simulink model "Simulation"  (R2020b)
settings: Solver=VariableStepAuto  StartTime=0.0  StopTime=10  RelTol=1e-3
undefined symbols (not defined in the file): Controller_Mode, DiscIntNeverNeededParam, InitalDroneXYZ, maxOmega, plant_N, ts_camera, ts_control
libraries: simulink x4, sim3dcameralib x3, uavsim3dlib x2, dspfdesign x1, rllib x1, deeplib x1, visiongeotforms x1, sim3dlib x1
settings Model: DataDictionary=Dictionary.sldd  EnableAccessToBaseWorkspace=off  VariantFading=off  OrderedModelArguments=off  Creator=elbit  LastModifiedBy=elbit
settings DebuggingCC: BusObjectLabelMismatch=error

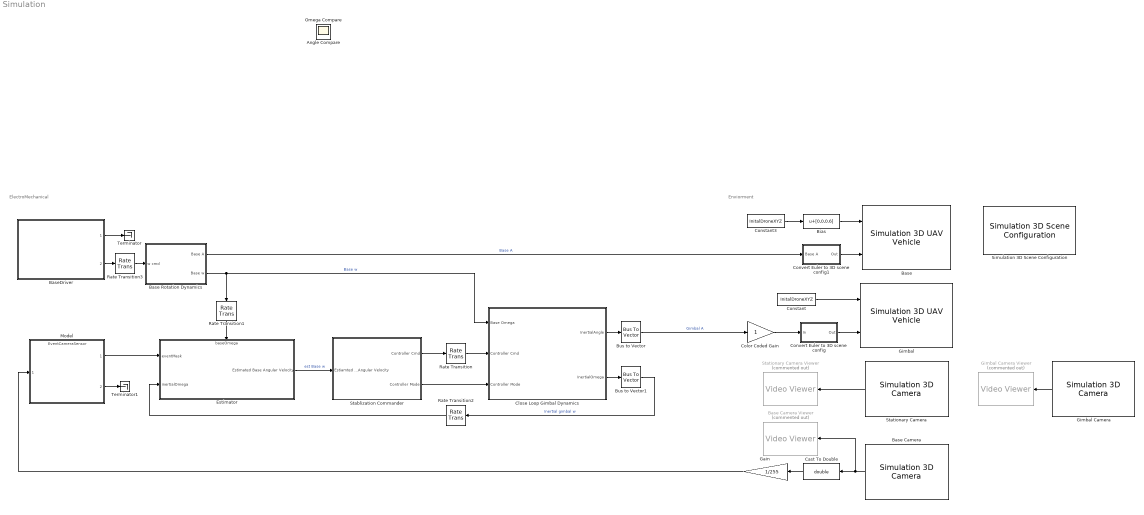
== system Simulation ==
  note: ElectroMechanical
  note: Enviorment
  Base : uavsim3dlib/Simulation 3D UAV Vehicle  Mesh=Quadrotor  Color=Black  ActorName=Base  InitialTranslation=InitalDroneXYZ  InitialRotation=[0 0 0]  SampleTime=-1  ActorType=SimulinkVehicle  ID=C  aMode=4  ActorTag=Base
      settings: SourceProductName=UAV Toolbox
  Base Camera : sim3dcameralib/Simulation 3D Camera  Priority=1  sensorTag=Sim3dSensor1  sensorId=1  sensorName=Sim3dSensor1  vehTagList={'Base';'Gimbal';'Scene Origin'}  vehTag=Base  mountLoc=Origin  offsetFlag=on  tmountOffset=[0.1, 0, 0]  rmountOffset=[0, 0, 0]  FocalLength=[1109, 1109]  OpticalCenter=[640, 360]  ImageSize=[720, 1280]  RadialDistortion=[0, 0]  TangentialDistortion=[0, 0]  SensorSkew=0  DepthOutportEnabled=off  SemanticOutportEnabled=off  TransformOutportEnabled=off  SampleTime=-1  mountPoint=[0.1 0 0]  mountOrientation=[0 0 0]  aMode=4  ID=1
      settings: SourceProductBaseCode=DR,UV,VE
  Base Camera Viewer : VideoViewer  Commented=on  FigPos=[2450.6 616.4 417.6 316]
  Base Rotation Dynamics : Subsystem  TreatAsAtomicUnit=on
  BaseDriver : Subsystem  TreatAsAtomicUnit=on  ReferencedSubsystem=BaseDriver
  Bias : Bias  Bias=[0,0,0.6]
  Bus to Vector : BusToVector
  Bus to Vector1 : BusToVector
  Cast To Double : DataTypeConversion  OutDataTypeStr=double
  Close Loop Gimbal Dynamics : Subsystem
  Color Coded Gain : Gain  OutDataTypeStr=Inherit: Same as input
      settings: OpenFcn=|
      | if get_param(gcbh,'gain')-48 set_param(gcbh,'gain','0','backgroundcolor','red');
      | else set_param(gcbh,'gain','1','backgroundcolor','green');
      | end
  Constant : Constant  Value=InitalDroneXYZ
  Constant3 : Constant  Value=InitalDroneXYZ
  Convert Euler to 3D scene config : Subsystem
  Convert Euler to 3D scene config1 : Subsystem
  Estimator : Subsystem  Variant=on  VariantControlMode=label  VariantControl=Choice  LabelModeActiveChoice=RNN
      settings: PortSchema="{\"entries\":[{\"content\":{\"sides\":[{\"content\":{\"connectorIds\":[\"In1\",\"In2\"]},\"type\":\"ConnectorPlacement.EquallySpacedRectSide\",\"uuid\":\"14ed0ca0-4e82-4a39-abac-b2cc8c23d388\"},{\"content\":{\"connectorIds\":[\"Out1\"],\"side\":\"RIGHT\"},\"type\":\"ConnectorPlacement.EquallySpacedRectSide\",\"uuid\":\"e489f507-16a0-46e9-ac1f-44f6d2c4c602\"},{\"content\":{\"connectorIds\":[\"In3\"],\"side\":\"TOP\"},\"type\":\"ConnectorPlacement.EquallySpacedRectSide\",\"uuid\":\"bc2047a9-ba61-4167-bd93-99be29e3b1d9\"},{\"content\":{\"connectorIds\":[],\"side\":\"HIDDEN\"},\"type\":\"ConnectorPlacement.EquallySpacedRectSide\",\"uuid\":\"51c71e1a-03eb-448f-a426-a7c596e1bf88\"}]},\"type\":\"ConnectorPlacement.EquallySpacedConnector\",\"uuid\":\"2c590113-b0cf-4c4b-9d58-bf60918ff368\"}],\"packageUris\":[\"http://schema.mathworks.com/mf0/Connector/R2020b\"],\"version\":\"1.0\"}"
  Gain : Gain  Gain=1/255
  Gimbal : uavsim3dlib/Simulation 3D UAV Vehicle  Mesh=Quadrotor  Color=Black  ActorName=Gimbal  InitialTranslation=InitalDroneXYZ  InitialRotation=[0 0 0]  SampleTime=-1  ActorType=SimulinkVehicle  ID=C  aMode=4  ActorTag=Gimbal
      settings: SourceProductName=UAV Toolbox
  Gimbal Camera : sim3dcameralib/Simulation 3D Camera  Priority=1  sensorTag=Sim3dSensor3  sensorId=3  sensorName=Sim3dSensor3  vehTagList={'Base';'Gimbal';'Scene Origin'}  vehTag=Gimbal  mountLoc=Origin  offsetFlag=on  tmountOffset=[0.1, 0, 0]  rmountOffset=[0, 0, 0]  FocalLength=[1109, 1109]  OpticalCenter=[640, 360]  ImageSize=[720, 1280]  RadialDistortion=[0, 0]  TangentialDistortion=[0, 0]  SensorSkew=0  DepthOutportEnabled=off  SemanticOutportEnabled=off  TransformOutportEnabled=off  SampleTime=-1  mountPoint=[0.1 0 0]  mountOrientation=[0 0 0]  aMode=4  ID=3
      settings: SourceProductBaseCode=DR,UV,VE
  Gimbal Camera Viewer : VideoViewer  Commented=on  FigPos=[125.8 875.6 524.8 320.8]
  Model : ModelReference  ModelNameDialog=EventCameraSensor.slx  ModelReferenceVersion=1.37
  Rate Transition : RateTransition  OutPortSampleTime=ts_control
  Rate Transition1 : RateTransition  OutPortSampleTime=ts_camera
  Rate Transition2 : RateTransition
  Rate Transition3 : RateTransition
  Simulation 3D Scene Configuration : sim3dlib/Simulation 3D Scene Configuration  Priority=0  ProjectFormat=Default Scenes  SceneDesc=US city block  ProjectName=MathWorks_Aerospace.exe  ScenePath=/Game/Maps/USCityBlock  vehTagList={'Base';'Gimbal';'Scene Origin'}  vehTag=Scene Origin  OpVisEn=off  Ts=ts_camera  EnableWindow=off  sensorTag=MainCamera1  sensorId=1  sensorName=MainCamera1  mountLoc=Origin  offsetFlag=off  tmountOffset=[0, 0, 0]  rmountOffset=[0, 0, 0]  HorizontalResolution=1280  VerticalResolution=720  HorizontalFOV=60  mountPoint=[0 0 0]  mountOrientation=[0 0 0]  aMode=4  ID=1
      settings: SourceProductBaseCode=DR,UV,VE
  Stablization Commander : Subsystem  TreatAsAtomicUnit=on
  Stationary Camera : sim3dcameralib/Simulation 3D Camera  Priority=1  sensorTag=Sim3dSensor2  sensorId=2  sensorName=Sim3dSensor2  vehTagList={'Base';'Gimbal';'Scene Origin'}  vehTag=Scene Origin  mountLoc=Origin  offsetFlag=on  tmountOffset=[10.88,83.6,8.181]  rmountOffset=[0,0.1047,-2.34]*180/pi  FocalLength=[1109, 1109]  OpticalCenter=[640, 360]  ImageSize=[720, 1280]  RadialDistortion=[0, 0]  TangentialDistortion=[0, 0]  SensorSkew=0  DepthOutportEnabled=off  SemanticOutportEnabled=off  TransformOutportEnabled=off  SampleTime=-1  mountPoint=[10.88 -83.6 8.181]  mountOrientation=[0 -5.99886811501972 134.072124060613]  aMode=4  ID=2
      settings: SourceProductBaseCode=DR,UV,VE
  Stationary Camera Viewer : VideoViewer  Commented=on  FigPos=[1048.2 851.6 517.6 520]
  Terminator : Terminator
  Terminator1 : Terminator
  Angle Compare : Scope
  Omega Compare : Scope
  wires:
  Constant/1 -> Gimbal/1
  Base Camera/1 -> Base Camera Viewer/1, Cast To Double/1
  Model/2 -> Terminator1/1
  Close Loop Gimbal Dynamics/1(InertialAngle) -> Bus to Vector/1
  Close Loop Gimbal Dynamics/2(InertialOmega) -> Bus to Vector1/1
  Cast To Double/1 -> Gain/1
  Gain/1 -> Model/1
  Bus to Vector/1 -> Color Coded Gain/1  "Gimbal A"
  Color Coded Gain/1 -> Convert Euler to 3D scene config/1(In)
  Stablization Commander/2(Controller Mode) -> Close Loop Gimbal Dynamics/3(Controller Mode)
  Stationary Camera/1 -> Stationary Camera Viewer/1
  Convert Euler to 3D scene config/1(Out) -> Gimbal/2
  Rate Transition1/1 -> Estimator/3(baseOmega)
  Rate Transition/1 -> Close Loop Gimbal Dynamics/2(Controller Cmd)
  Stablization Commander/1(Controller Cmd) -> Rate Transition/1
  Convert Euler to 3D scene config1/1(Out) -> Base/2
  Constant3/1 -> Bias/1
  Base Rotation Dynamics/1(Base A) -> Convert Euler to 3D scene config1/1(Base A)  "Base A"
  Bus to Vector1/1 -> Rate Transition2/1  "Inertial gimbal w"
  Bias/1 -> Base/1
  BaseDriver/2 -> Rate Transition3/1
  BaseDriver/1 -> Terminator/1
  Model/1 -> Estimator/1(eventMask)
  Base Rotation Dynamics/2(Base w) -> Close Loop Gimbal Dynamics/1(Base Omega), Rate Transition1/1  "Base w"
  Gimbal Camera/1 -> Gimbal Camera Viewer/1
  Rate Transition2/1 -> Estimator/2(inertialOmega)
  Rate Transition3/1 -> Base Rotation Dynamics/1(w cmd)
  Estimator/1(Estimated Base Angular Velocity) -> Stablization Commander/1(Estiamted Base Angular Velocity)  "est Base w"

== system Simulation/Base Rotation Dynamics ==
  w cmd : Inport
  Demux : Demux  Outputs=3
  Mux : Mux  Inputs=3
  RotationIntegrator : Integrator  InitialCondition=[0 0 0]
  Transfer Fcn : TransferFcn  Numerator=(2*pi*7)^2  Denominator=[1,2*1*(2*pi*7),(2*pi*7)^2]
  Transfer Fcn1 : TransferFcn  Numerator=(2*pi*7)^2  Denominator=[1,2*1*(2*pi*7),(2*pi*7)^2]
  Transfer Fcn2 : TransferFcn  Numerator=(2*pi*7)^2  Denominator=[1,2*1*(2*pi*7),(2*pi*7)^2]
  Base A : Outport
  Base w : Outport  Port=2
  wires:
  Demux/3 -> Transfer Fcn2/1
  Demux/2 -> Transfer Fcn1/1
  RotationIntegrator/1 -> Base A/1
  w cmd/1 -> Demux/1
  Mux/1 -> Base w/1, RotationIntegrator/1
  Transfer Fcn2/1 -> Mux/3
  Transfer Fcn1/1 -> Mux/2
  Transfer Fcn/1 -> Mux/1
  Demux/1 -> Transfer Fcn/1

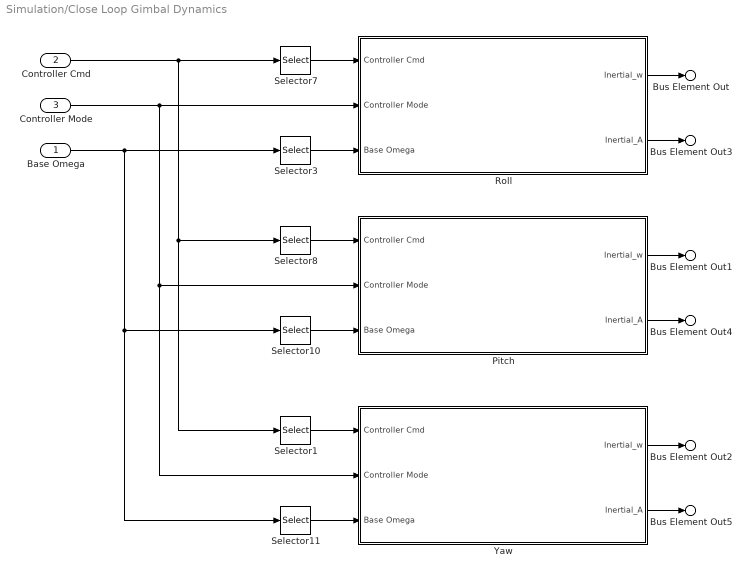
== system Simulation/Close Loop Gimbal Dynamics ==
  Base Omega : Inport
  Controller Cmd : Inport  Port=2
  Controller Mode : Inport  Port=3
  Pitch : Subsystem  Variant=on  VariantControlMode=label  VariantControl=Choice  LabelModeActiveChoice=Simple
  Roll : Subsystem  Variant=on  VariantControlMode=label  VariantControl=Choice  LabelModeActiveChoice=Simple
  Selector1 : Selector  InputPortWidth=3  IndexOptions=Index vector (dialog)  Indices=3  OutputSizes=1
  Selector10 : Selector  InputPortWidth=3  IndexOptions=Index vector (dialog)  Indices=2  OutputSizes=1
  Selector11 : Selector  InputPortWidth=3  IndexOptions=Index vector (dialog)  Indices=3  OutputSizes=1
  Selector3 : Selector  InputPortWidth=3  IndexOptions=Index vector (dialog)  Indices=1  OutputSizes=1
  Selector7 : Selector  InputPortWidth=3  IndexOptions=Index vector (dialog)  Indices=1  OutputSizes=1
  Selector8 : Selector  InputPortWidth=3  IndexOptions=Index vector (dialog)  Indices=2  OutputSizes=1
  Yaw : Subsystem  Variant=on  VariantControlMode=label  VariantControl=Choice  LabelModeActiveChoice=Simple
  Bus Element Out3 : Outport  PortName=InertialAngle  Element=Roll
  Bus Element Out4 : Outport  PortName=InertialAngle  Element=Pitch
  Bus Element Out5 : Outport  PortName=InertialAngle  Element=Yaw
  Bus Element Out : Outport  Port=2  PortName=InertialOmega  Element=Roll
  Bus Element Out1 : Outport  Port=2  PortName=InertialOmega  Element=Pitch
  Bus Element Out2 : Outport  Port=2  PortName=InertialOmega  Element=Yaw
  wires:
  Pitch/1(Inertial_w) -> Bus Element Out1/1
  Yaw/1(Inertial_w) -> Bus Element Out2/1
  Pitch/2(Inertial_A) -> Bus Element Out4/1
  Yaw/2(Inertial_A) -> Bus Element Out5/1
  Selector8/1 -> Pitch/1(Controller Cmd)
  Controller Cmd/1 -> Selector1/1, Selector8/1, Selector7/1
  Base Omega/1 -> Selector11/1, Selector10/1, Selector3/1
  Selector10/1 -> Pitch/3(Base Omega)
  Selector1/1 -> Yaw/1(Controller Cmd)
  Selector11/1 -> Yaw/3(Base Omega)
  Controller Mode/1 -> Roll/2(Controller Mode), Yaw/2(Controller Mode), Pitch/2(Controller Mode)
  Selector7/1 -> Roll/1(Controller Cmd)
  Selector3/1 -> Roll/3(Base Omega)
  Roll/1(Inertial_w) -> Bus Element Out/1
  Roll/2(Inertial_A) -> Bus Element Out3/1

== system Simulation/Convert Euler to 3D scene config ==
  In : Inport
  Mux : Mux  Inputs=3
  Selector : Selector  InputPortWidth=3  IndexOptions=Index vector (dialog)  Indices=1  OutputSizes=1
  Selector1 : Selector  InputPortWidth=3  IndexOptions=Index vector (dialog)  Indices=2  OutputSizes=1
  Selector2 : Selector  InputPortWidth=3  IndexOptions=Index vector (dialog)  Indices=3  OutputSizes=1
  Out : Outport
  wires:
  Mux/1 -> Out/1
  Selector1/1 -> Mux/2
  Selector/1 -> Mux/3
  In/1 -> Selector/1, Selector1/1, Selector2/1
  Selector2/1 -> Mux/1

== system Simulation/Convert Euler to 3D scene config1 ==
  Base A : Inport
  Mux : Mux  Inputs=3
  Selector : Selector  InputPortWidth=3  IndexOptions=Index vector (dialog)  Indices=1  OutputSizes=1
  Selector1 : Selector  InputPortWidth=3  IndexOptions=Index vector (dialog)  Indices=2  OutputSizes=1
  Selector2 : Selector  InputPortWidth=3  IndexOptions=Index vector (dialog)  Indices=3  OutputSizes=1
  Out : Outport
  wires:
  Selector2/1 -> Mux/1
  Base A/1 -> Selector2/1, Selector1/1, Selector/1
  Selector/1 -> Mux/3
  Selector1/1 -> Mux/2
  Mux/1 -> Out/1

== system Simulation/Estimator ==
  eventMask : Inport
  inertialOmega : Inport  Port=2
  baseOmega : Inport  Port=3
  GroundTruth : Subsystem  TreatAsAtomicUnit=on  VariantControl=GroundTruth
  RL : Subsystem  TreatAsAtomicUnit=on  VariantControl=RL
  RNN : Subsystem  TreatAsAtomicUnit=on  VariantControl=RNN
  Estimated Base Angular Velocity : Outport

== system Simulation/Stablization Commander ==
  Estiamted Base Angular Velocity : Inport
  Enumerated Constant : simulink/Sources/Enumerated Constant  OutDataTypeStr=Enum: Controller_Mode  Value=Controller_Mode.Velocity  SampleTime=inf
  Load2MotorVel : Gain  Gain=plant_N
  Unary Minus : UnaryMinus
  Controller Cmd : Outport
  Controller Mode : Outport  Port=2
  wires:
  Enumerated Constant/1 -> Controller Mode/1
  Estiamted Base Angular Velocity/1 -> Unary Minus/1
  Unary Minus/1 -> Load2MotorVel/1
  Load2MotorVel/1 -> Controller Cmd/1

== system Simulation/Close Loop Gimbal Dynamics/Pitch ==
  Controller Cmd : Inport
  Controller Mode : Inport  Port=2
  Base Omega : Inport  Port=3
  Complex : Subsystem  VariantControl=Complex
  Simple : Subsystem  TreatAsAtomicUnit=on  VariantControl=Simple
  Inertial_w : Outport
  Inertial_A : Outport  Port=2

== system Simulation/Close Loop Gimbal Dynamics/Roll ==
  Controller Cmd : Inport
  Controller Mode : Inport  Port=2
  Base Omega : Inport  Port=3
  Complex : Subsystem  VariantControl=Complex
  Simple : Subsystem  TreatAsAtomicUnit=on  VariantControl=Simple
  Inertial_w : Outport
  Inertial_A : Outport  Port=2

== system Simulation/Close Loop Gimbal Dynamics/Yaw ==
  Controller Cmd : Inport
  Controller Mode : Inport  Port=2
  Base Omega : Inport  Port=3
  Complex : Subsystem  VariantControl=Complex
  Simple : Subsystem  TreatAsAtomicUnit=on  VariantControl=Simple
  Inertial_w : Outport
  Inertial_A : Outport  Port=2

== system Simulation/Estimator/GroundTruth ==
  baseOmega : Inport
  Estimated Base Angular Velocity : Outport
  wires:
  baseOmega/1 -> Estimated Base Angular Velocity/1

== system Simulation/Estimator/RL ==
  eventMask : Inport
  inertialOmega : Inport  Port=2
  CalcualteReward : Subsystem
  Constant : Constant  Value=0  OutDataTypeStr=boolean
  Demux : Demux  Outputs=3
  Mux : Mux  Inputs=3
  RL Agent : rllib/RL Agent  Agent=rlAgent  ProvideReward=on  ProvideIsDone=on  ProvideCumRwd=off  TreatAsDirectFeedthrough=on  CollectLoggedSignals=on  CollectModelStates=on
  Saturation : Saturate  UpperLimit=maxOmega  LowerLimit=-maxOmega
  Estimated Base Angular Velocity : Outport
  wires:
  eventMask/1 -> RL Agent/1
  Saturation/1 -> Estimated Base Angular Velocity/1, CalcualteReward/2(EstimatedOmega)
  Constant/1 -> RL Agent/3
  inertialOmega/1 -> CalcualteReward/1(InertialOmega)
  CalcualteReward/1(reward) -> RL Agent/2
  Demux/1 -> Mux/1
  Demux/2 -> Mux/2
  Demux/3 -> Mux/3
  RL Agent/1 -> Demux/1
  Mux/1 -> Saturation/1

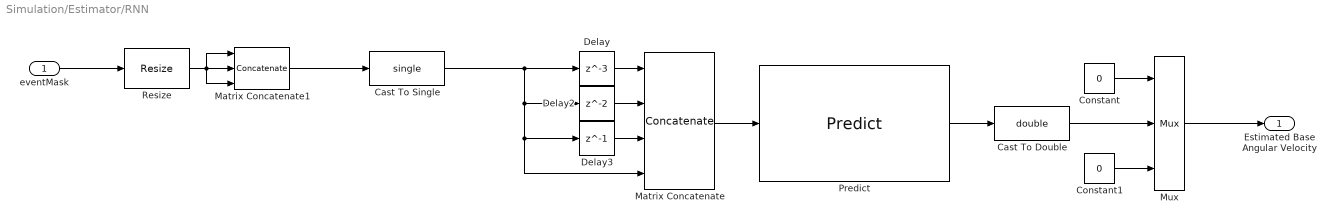
== system Simulation/Estimator/RNN ==
  eventMask : Inport
  Cast To Double : DataTypeConversion  OutDataTypeStr=double
  Cast To Single : DataTypeConversion  OutDataTypeStr=single
  Constant : Constant  Value=0
  Constant1 : Constant  Value=0
  Delay : Delay  DelayLength=3
  Delay2 : Delay
  Delay3 : Delay  DelayLength=1
  Matrix Concatenate : Concatenate  NumInputs=4  Mode=Multidimensional array  ConcatenateDimension=4
  Matrix Concatenate1 : Concatenate  NumInputs=3  Mode=Multidimensional array  ConcatenateDimension=3
  Mux : Mux  Inputs=3
  Predict : deeplib/Predict  Network=Network from MAT-file  NetworkFunction=squeezenet  NetworkFilePath=C:\Users\elbit\Desktop\Technion\EventCameraStablization\DeepLearning\E2wNet.mat  MiniBatchSize=1  InputDataFormats={ '', '' }  Predictions=on  Activations={}  ForceInterpretedSim=off  EnableDLNetwork=off
      settings: SourceProductBaseCode=NN
  Resize : visiongeotforms/Resize  specify=Number of output rows and columns  rfactor=[]  outCols=25  outRows=25  outRowsCols=[244 244]  interp_method=Bilinear  antialias=on  useROI=off  roiFlag=off  roundingMode=Nearest  overflowMode=on  prodOutputMode=Binary point scaling  prodOutputWordLength=32  prodOutputFracLength=10
      settings: SourceProductBaseCode=VP
  Estimated Base Angular Velocity : Outport
  wires:
  Predict/1 -> Cast To Double/1
  eventMask/1 -> Resize/1
  Delay/1 -> Matrix Concatenate/1
  Delay2/1 -> Matrix Concatenate/2
  Delay3/1 -> Matrix Concatenate/3
  Cast To Single/1 -> Delay/1, Delay2/1, Delay3/1, Matrix Concatenate/4
  Matrix Concatenate/1 -> Predict/1
  Matrix Concatenate1/1 -> Cast To Single/1
  Resize/1 -> Matrix Concatenate1/1, Matrix Concatenate1/2, Matrix Concatenate1/3
  Cast To Double/1 -> Mux/2
  Constant/1 -> Mux/1
  Constant1/1 -> Mux/3
  Mux/1 -> Estimated Base Angular Velocity/1

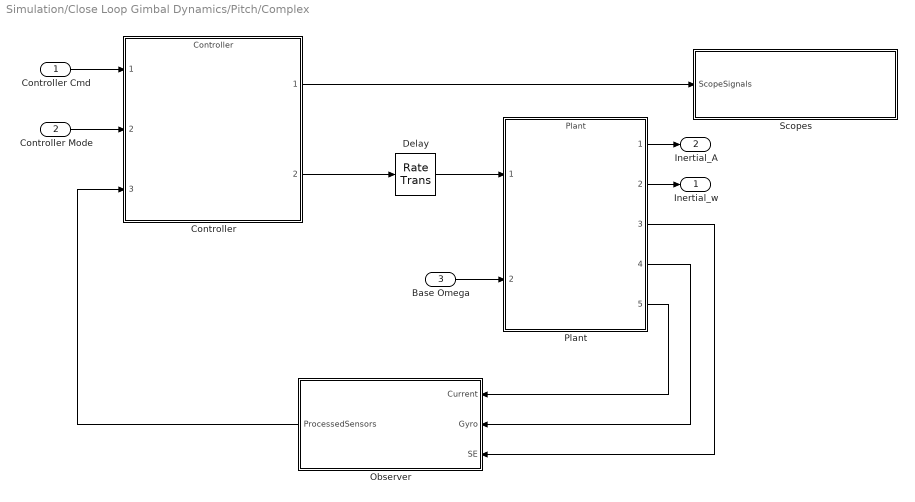
== system Simulation/Close Loop Gimbal Dynamics/Pitch/Complex ==
  Controller Cmd : Inport
  Controller Mode : Inport  Port=2
  Base Omega : Inport  Port=3
  Controller : ModelReference  ModelNameDialog=Controller  SimulationMode=Normal  ModelReferenceVersion=1.79
  Delay : RateTransition  OutPortSampleTime=0
  Observer : Subsystem  TreatAsAtomicUnit=on
  Plant : ModelReference  ModelNameDialog=Plant  ModelReferenceVersion=1.81
  Scopes : Subsystem
  Inertial_w : Outport
  Inertial_A : Outport  Port=2
  wires:
  Controller/1 -> Scopes/1(ScopeSignals)
  Controller/2 -> Delay/1
  Base Omega/1 -> Plant/2
  Plant/2 -> Inertial_w/1
  Plant/3 -> Observer/3(SE)
  Plant/4 -> Observer/2(Gyro)
  Plant/5 -> Observer/1(Current)
  Observer/1(ProcessedSensors) -> Controller/3
  Controller Mode/1 -> Controller/2
  Delay/1 -> Plant/1
  Controller Cmd/1 -> Controller/1
  Plant/1 -> Inertial_A/1

== system Simulation/Close Loop Gimbal Dynamics/Pitch/Simple ==
  Controller Cmd : Inport
  Base Omega : Inport  Port=2
  Closed Vel Loop : Subsystem
  Integrator : Integrator
  Integrator1 : Integrator
  Sum : Sum  Inputs=|++
  Sum1 : Sum  Inputs=|++
  Inertial_w : Outport
  Inertial_A : Outport  Port=2
  wires:
  Controller Cmd/1 -> Closed Vel Loop/1(Relative_w_cmd)
  Closed Vel Loop/1(Relative_w) -> Sum/1, Integrator/1
  Sum1/1 -> Inertial_A/1
  Integrator1/1 -> Sum1/2  "Base_w"
  Integrator/1 -> Sum1/1  "Relative_A"
  Sum/1 -> Inertial_w/1
  Base Omega/1 -> Sum/2, Integrator1/1

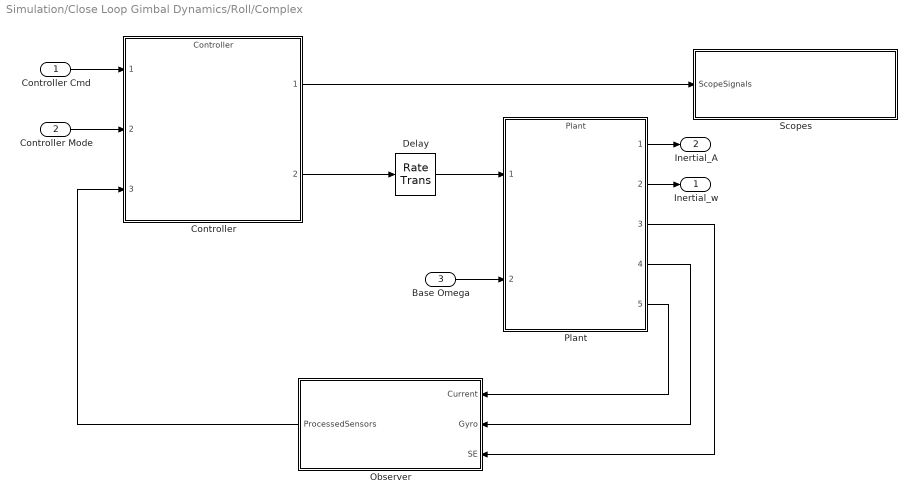
== system Simulation/Close Loop Gimbal Dynamics/Roll/Complex ==
  Controller Cmd : Inport
  Controller Mode : Inport  Port=2
  Base Omega : Inport  Port=3
  Controller : ModelReference  ModelNameDialog=Controller  SimulationMode=Normal  ModelReferenceVersion=1.79
  Delay : RateTransition  OutPortSampleTime=0
  Observer : Subsystem  TreatAsAtomicUnit=on
  Plant : ModelReference  ModelNameDialog=Plant  ModelReferenceVersion=1.81
  Scopes : Subsystem
  Inertial_w : Outport
  Inertial_A : Outport  Port=2
  wires:
  Plant/1 -> Inertial_A/1
  Controller Cmd/1 -> Controller/1
  Delay/1 -> Plant/1
  Controller Mode/1 -> Controller/2
  Observer/1(ProcessedSensors) -> Controller/3
  Plant/5 -> Observer/1(Current)
  Plant/4 -> Observer/2(Gyro)
  Plant/3 -> Observer/3(SE)
  Plant/2 -> Inertial_w/1
  Base Omega/1 -> Plant/2
  Controller/2 -> Delay/1
  Controller/1 -> Scopes/1(ScopeSignals)

== system Simulation/Close Loop Gimbal Dynamics/Roll/Simple ==
  Controller Cmd : Inport
  Base Omega : Inport  Port=2
  Closed Vel Loop : Subsystem
  Integrator : Integrator
  Integrator1 : Integrator
  Sum : Sum  Inputs=|++
  Sum1 : Sum  Inputs=|++
  Inertial_w : Outport
  Inertial_A : Outport  Port=2
  wires:
  Base Omega/1 -> Integrator1/1, Sum/2
  Sum/1 -> Inertial_w/1
  Integrator/1 -> Sum1/1  "Relative_A"
  Integrator1/1 -> Sum1/2  "Base_w"
  Sum1/1 -> Inertial_A/1
  Closed Vel Loop/1(Relative_w) -> Integrator/1, Sum/1
  Controller Cmd/1 -> Closed Vel Loop/1(Relative_w_cmd)

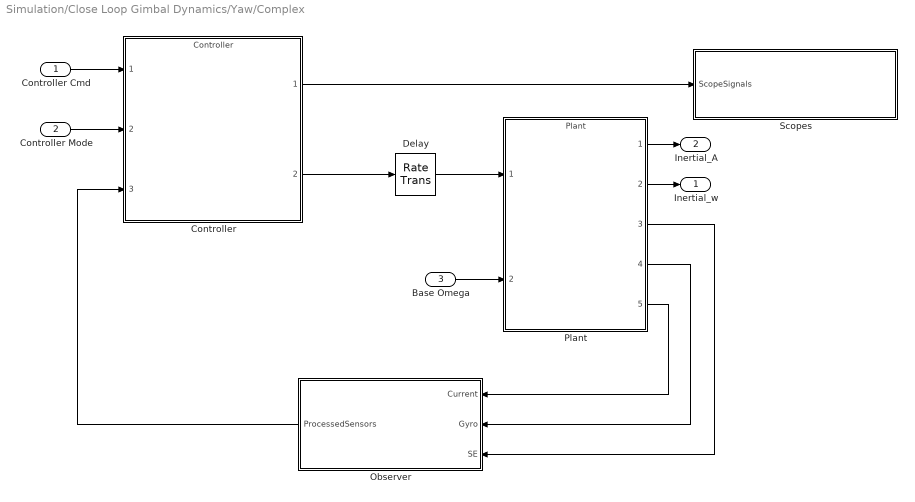
== system Simulation/Close Loop Gimbal Dynamics/Yaw/Complex ==
  Controller Cmd : Inport
  Controller Mode : Inport  Port=2
  Base Omega : Inport  Port=3
  Controller : ModelReference  ModelNameDialog=Controller  SimulationMode=Normal  ModelReferenceVersion=1.79
  Delay : RateTransition  OutPortSampleTime=0
  Observer : Subsystem  TreatAsAtomicUnit=on
  Plant : ModelReference  ModelNameDialog=Plant  ModelReferenceVersion=1.81
  Scopes : Subsystem
  Inertial_w : Outport
  Inertial_A : Outport  Port=2
  wires:
  Plant/1 -> Inertial_A/1
  Controller Cmd/1 -> Controller/1
  Delay/1 -> Plant/1
  Controller Mode/1 -> Controller/2
  Observer/1(ProcessedSensors) -> Controller/3
  Plant/5 -> Observer/1(Current)
  Plant/4 -> Observer/2(Gyro)
  Plant/3 -> Observer/3(SE)
  Plant/2 -> Inertial_w/1
  Base Omega/1 -> Plant/2
  Controller/2 -> Delay/1
  Controller/1 -> Scopes/1(ScopeSignals)

== system Simulation/Close Loop Gimbal Dynamics/Yaw/Simple ==
  Controller Cmd : Inport
  Base Omega : Inport  Port=2
  Closed Vel Loop : Subsystem
  Integrator : Integrator
  Integrator1 : Integrator
  Sum : Sum  Inputs=|++
  Sum1 : Sum  Inputs=|++
  Inertial_w : Outport
  Inertial_A : Outport  Port=2
  wires:
  Base Omega/1 -> Integrator1/1, Sum/2
  Sum/1 -> Inertial_w/1
  Integrator/1 -> Sum1/1  "Relative_A"
  Integrator1/1 -> Sum1/2  "Base_w"
  Sum1/1 -> Inertial_A/1
  Closed Vel Loop/1(Relative_w) -> Integrator/1, Sum/1
  Controller Cmd/1 -> Closed Vel Loop/1(Relative_w_cmd)

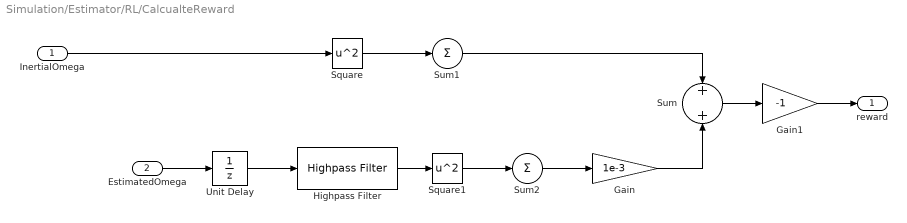
== system Simulation/Estimator/RL/CalcualteReward ==
  InertialOmega : Inport
  EstimatedOmega : Inport  Port=2
  Gain : Gain  Gain=1e-3
  Gain1 : Gain  Gain=-1
  Highpass Filter : dspfdesign/Highpass Filter  FilterType=FIR  DesignForMinimumOrder=on  FilterOrder=50  StopbandFrequency=10  PassbandFrequency=20  StopbandAttenuation=40  PassbandRipple=0.1  InheritSampleRate=off  SampleRate=1/ts_camera  SimulateUsing=Interpreted execution  roundingMode=Floor  coeffsDataTypeStr=fixdt(1,16)
  Square : Math  Operator=square  SaturateOnIntegerOverflow=on
  Square1 : Math  Operator=square  SaturateOnIntegerOverflow=on
  Sum : Sum
  Sum1 : Sum  Inputs=+
  Sum2 : Sum  Inputs=+
  Unit Delay : UnitDelay  SampleTime=-1  HasFrameUpgradeWarning=on
  reward : Outport
  wires:
  InertialOmega/1 -> Square/1
  Unit Delay/1 -> Highpass Filter/1
  EstimatedOmega/1 -> Unit Delay/1
  Highpass Filter/1 -> Square1/1
  Gain/1 -> Sum/2
  Square/1 -> Sum1/1
  Sum/1 -> Gain1/1
  Gain1/1 -> reward/1
  Sum1/1 -> Sum/1
  Sum2/1 -> Gain/1
  Square1/1 -> Sum2/1

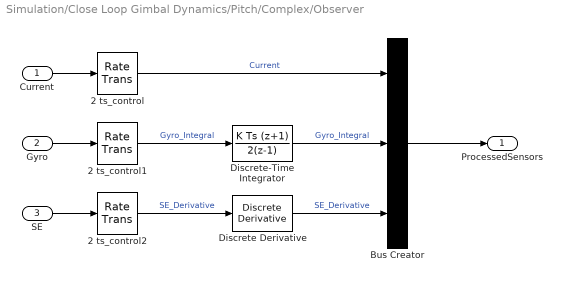
== system Simulation/Close Loop Gimbal Dynamics/Pitch/Complex/Observer ==
  Current : Inport  SampleTime=ts_control
  Gyro : Inport  Port=2  SampleTime=ts_control
  SE : Inport  Port=3  SampleTime=ts_control
  2 ts_control : RateTransition  OutPortSampleTime=ts_control
  2 ts_control1 : RateTransition  OutPortSampleTime=ts_control
  2 ts_control2 : RateTransition  OutPortSampleTime=ts_control
  Bus Creator : BusCreator  Inputs=3  OutDataTypeStr=Bus: Processed_Sensors
  Discrete Derivative : simulink/Discrete/Discrete Derivative  gainval=1.0  ICPrevScaledInput=0.0  OutMin=[]  OutMax=[]  OutDataType=fixdt(1, 16)  OutScaling=2^-10  DoSatur=off
  Discrete-Time Integrator : DiscreteIntegrator  IntegratorMethod=Integration: Trapezoidal  SampleTime=-1  ICPrevOutput=DiscIntNeverNeededParam  ICPrevScaledInput=DiscIntNeverNeededParam
  ProcessedSensors : Outport  OutDataTypeStr=Bus: Processed_Sensors  SampleTime=ts_control
  wires:
  2 ts_control/1 -> Bus Creator/1  "Current"
  Current/1 -> 2 ts_control/1
  SE/1 -> 2 ts_control2/1
  2 ts_control2/1 -> Discrete Derivative/1  "SE_Derivative"
  Gyro/1 -> 2 ts_control1/1
  2 ts_control1/1 -> Discrete-Time Integrator/1  "Gyro_Integral"
  Discrete-Time Integrator/1 -> Bus Creator/2  "Gyro_Integral"
  Discrete Derivative/1 -> Bus Creator/3  "SE_Derivative"
  Bus Creator/1 -> ProcessedSensors/1

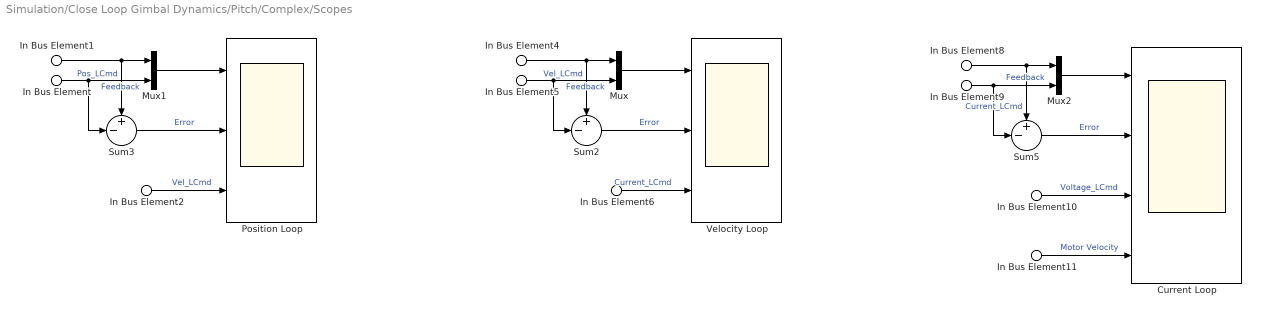
== system Simulation/Close Loop Gimbal Dynamics/Pitch/Complex/Scopes ==
  In Bus Element : Inport  PortName=ScopeSignals  Element=Position.Gyro_Integral
  In Bus Element1 : Inport  PortName=ScopeSignals  Element=Position.Pos_LCmd
  In Bus Element2 : Inport  PortName=ScopeSignals  Element=Position.Vel_LCmd
  In Bus Element4 : Inport  PortName=ScopeSignals  Element=Velocity.Vel_LCmd
  In Bus Element5 : Inport  PortName=ScopeSignals  Element=Velocity.SE_Derivative
  In Bus Element6 : Inport  PortName=ScopeSignals  Element=Velocity.Current_LCmd
  In Bus Element8 : Inport  PortName=ScopeSignals  Element=Current.Current_LCmd
  In Bus Element9 : Inport  PortName=ScopeSignals  Element=Current.Current
  In Bus Element10 : Inport  PortName=ScopeSignals  Element=Current.Voltage_LCmd
  In Bus Element11 : Inport  PortName=ScopeSignals  Element=Current.SE_Derivative
  Current Loop : Scope  NumInputPorts=4
  Mux : Mux  Inputs=2
  Mux1 : Mux  Inputs=2
  Mux2 : Mux  Inputs=2
  Position Loop : Scope  NumInputPorts=3
  Sum2 : Sum  Inputs=+-|
  Sum3 : Sum  Inputs=+-|
  Sum5 : Sum  Inputs=+-|
  Velocity Loop : Scope  NumInputPorts=3
  wires:
  Sum2/1 -> Velocity Loop/2  "Error"
  In Bus Element4/1 -> Mux/1, Sum2/1  "Vel_LCmd"
  Sum3/1 -> Position Loop/2  "Error"
  Mux1/1 -> Position Loop/1
  In Bus Element6/1 -> Velocity Loop/3  "Current_LCmd"
  Mux/1 -> Velocity Loop/1
  In Bus Element1/1 -> Mux1/1, Sum3/1  "Pos_LCmd"
  In Bus Element5/1 -> Mux/2, Sum2/2  "Feedback"
  In Bus Element11/1 -> Current Loop/4  "Motor Velocity"
  In Bus Element9/1 -> Mux2/2, Sum5/2  "Feedback"
  Mux2/1 -> Current Loop/1
  In Bus Element2/1 -> Position Loop/3  "Vel_LCmd"
  In Bus Element10/1 -> Current Loop/3  "Voltage_LCmd"
  Sum5/1 -> Current Loop/2  "Error"
  In Bus Element8/1 -> Mux2/1, Sum5/1  "Current_LCmd"
  In Bus Element/1 -> Mux1/2, Sum3/2  "Feedback"

== system Simulation/Close Loop Gimbal Dynamics/Pitch/Simple/Closed Vel Loop ==
  Relative_w_cmd : Inport
  Closed Vel Loop1 : TransferFcn  Denominator=[1/(2*pi*15) 1]
  Closed Vel Loop2 : Integrator
  Gain : Gain  Gain=db2mag(42)
  Motor2Load : Gain  Gain=1/plant_N
  Sum2 : Sum  Inputs=|+-
  Relative_w : Outport
  wires:
  Gain/1 -> Closed Vel Loop1/1
  Sum2/1 -> Gain/1
  Closed Vel Loop2/1 -> Sum2/2, Relative_w/1  "Relative_w"
  Closed Vel Loop1/1 -> Closed Vel Loop2/1
  Motor2Load/1 -> Sum2/1
  Relative_w_cmd/1 -> Motor2Load/1

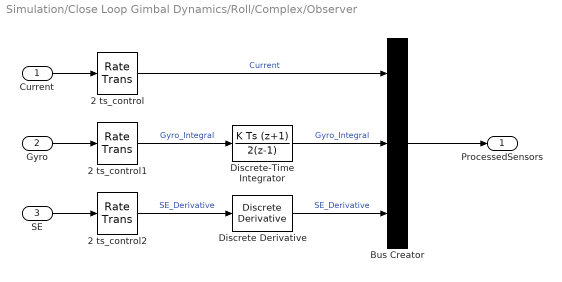
== system Simulation/Close Loop Gimbal Dynamics/Roll/Complex/Observer ==
  Current : Inport  SampleTime=ts_control
  Gyro : Inport  Port=2  SampleTime=ts_control
  SE : Inport  Port=3  SampleTime=ts_control
  2 ts_control : RateTransition  OutPortSampleTime=ts_control
  2 ts_control1 : RateTransition  OutPortSampleTime=ts_control
  2 ts_control2 : RateTransition  OutPortSampleTime=ts_control
  Bus Creator : BusCreator  Inputs=3  OutDataTypeStr=Bus: Processed_Sensors
  Discrete Derivative : simulink/Discrete/Discrete Derivative  gainval=1.0  ICPrevScaledInput=0.0  OutMin=[]  OutMax=[]  OutDataType=fixdt(1, 16)  OutScaling=2^-10  DoSatur=off
  Discrete-Time Integrator : DiscreteIntegrator  IntegratorMethod=Integration: Trapezoidal  SampleTime=-1  ICPrevOutput=DiscIntNeverNeededParam  ICPrevScaledInput=DiscIntNeverNeededParam
  ProcessedSensors : Outport  OutDataTypeStr=Bus: Processed_Sensors  SampleTime=ts_control
  wires:
  Bus Creator/1 -> ProcessedSensors/1
  Discrete Derivative/1 -> Bus Creator/3  "SE_Derivative"
  Discrete-Time Integrator/1 -> Bus Creator/2  "Gyro_Integral"
  2 ts_control1/1 -> Discrete-Time Integrator/1  "Gyro_Integral"
  Gyro/1 -> 2 ts_control1/1
  2 ts_control2/1 -> Discrete Derivative/1  "SE_Derivative"
  SE/1 -> 2 ts_control2/1
  Current/1 -> 2 ts_control/1
  2 ts_control/1 -> Bus Creator/1  "Current"

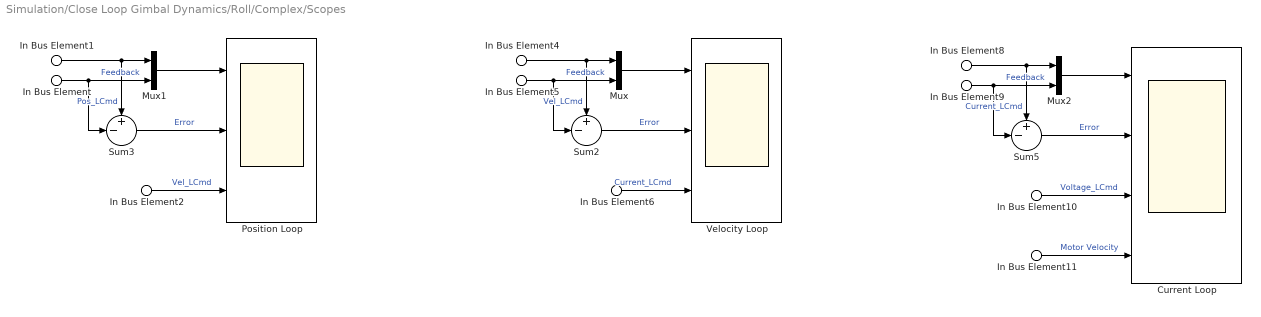
== system Simulation/Close Loop Gimbal Dynamics/Roll/Complex/Scopes ==
  In Bus Element : Inport  PortName=ScopeSignals  Element=Position.Gyro_Integral
  In Bus Element1 : Inport  PortName=ScopeSignals  Element=Position.Pos_LCmd
  In Bus Element2 : Inport  PortName=ScopeSignals  Element=Position.Vel_LCmd
  In Bus Element4 : Inport  PortName=ScopeSignals  Element=Velocity.Vel_LCmd
  In Bus Element5 : Inport  PortName=ScopeSignals  Element=Velocity.SE_Derivative
  In Bus Element6 : Inport  PortName=ScopeSignals  Element=Velocity.Current_LCmd
  In Bus Element8 : Inport  PortName=ScopeSignals  Element=Current.Current_LCmd
  In Bus Element9 : Inport  PortName=ScopeSignals  Element=Current.Current
  In Bus Element10 : Inport  PortName=ScopeSignals  Element=Current.Voltage_LCmd
  In Bus Element11 : Inport  PortName=ScopeSignals  Element=Current.SE_Derivative
  Current Loop : Scope  NumInputPorts=4
  Mux : Mux  Inputs=2
  Mux1 : Mux  Inputs=2
  Mux2 : Mux  Inputs=2
  Position Loop : Scope  NumInputPorts=3
  Sum2 : Sum  Inputs=+-|
  Sum3 : Sum  Inputs=+-|
  Sum5 : Sum  Inputs=+-|
  Velocity Loop : Scope  NumInputPorts=3
  wires:
  In Bus Element/1 -> Sum3/2, Mux1/2  "Feedback"
  In Bus Element8/1 -> Sum5/1, Mux2/1  "Current_LCmd"
  Sum5/1 -> Current Loop/2  "Error"
  In Bus Element10/1 -> Current Loop/3  "Voltage_LCmd"
  In Bus Element2/1 -> Position Loop/3  "Vel_LCmd"
  Mux2/1 -> Current Loop/1
  In Bus Element9/1 -> Sum5/2, Mux2/2  "Feedback"
  In Bus Element11/1 -> Current Loop/4  "Motor Velocity"
  In Bus Element5/1 -> Sum2/2, Mux/2  "Feedback"
  In Bus Element1/1 -> Sum3/1, Mux1/1  "Pos_LCmd"
  Mux/1 -> Velocity Loop/1
  In Bus Element6/1 -> Velocity Loop/3  "Current_LCmd"
  Mux1/1 -> Position Loop/1
  Sum3/1 -> Position Loop/2  "Error"
  In Bus Element4/1 -> Sum2/1, Mux/1  "Vel_LCmd"
  Sum2/1 -> Velocity Loop/2  "Error"

== system Simulation/Close Loop Gimbal Dynamics/Roll/Simple/Closed Vel Loop ==
  Relative_w_cmd : Inport
  Closed Vel Loop1 : TransferFcn  Denominator=[1/(2*pi*15) 1]
  Closed Vel Loop2 : Integrator
  Gain : Gain  Gain=db2mag(42)
  Motor2Load : Gain  Gain=1/plant_N
  Sum2 : Sum  Inputs=|+-
  Relative_w : Outport
  wires:
  Relative_w_cmd/1 -> Motor2Load/1
  Motor2Load/1 -> Sum2/1
  Closed Vel Loop1/1 -> Closed Vel Loop2/1
  Closed Vel Loop2/1 -> Relative_w/1, Sum2/2  "Relative_w"
  Sum2/1 -> Gain/1
  Gain/1 -> Closed Vel Loop1/1

== system Simulation/Close Loop Gimbal Dynamics/Yaw/Complex/Observer ==
  Current : Inport  SampleTime=ts_control
  Gyro : Inport  Port=2  SampleTime=ts_control
  SE : Inport  Port=3  SampleTime=ts_control
  2 ts_control : RateTransition  OutPortSampleTime=ts_control
  2 ts_control1 : RateTransition  OutPortSampleTime=ts_control
  2 ts_control2 : RateTransition  OutPortSampleTime=ts_control
  Bus Creator : BusCreator  Inputs=3  OutDataTypeStr=Bus: Processed_Sensors
  Discrete Derivative : simulink/Discrete/Discrete Derivative  gainval=1.0  ICPrevScaledInput=0.0  OutMin=[]  OutMax=[]  OutDataType=fixdt(1, 16)  OutScaling=2^-10  DoSatur=off
  Discrete-Time Integrator : DiscreteIntegrator  IntegratorMethod=Integration: Trapezoidal  SampleTime=-1  ICPrevOutput=DiscIntNeverNeededParam  ICPrevScaledInput=DiscIntNeverNeededParam
  ProcessedSensors : Outport  OutDataTypeStr=Bus: Processed_Sensors  SampleTime=ts_control
  wires:
  Bus Creator/1 -> ProcessedSensors/1
  Discrete Derivative/1 -> Bus Creator/3  "SE_Derivative"
  Discrete-Time Integrator/1 -> Bus Creator/2  "Gyro_Integral"
  2 ts_control1/1 -> Discrete-Time Integrator/1  "Gyro_Integral"
  Gyro/1 -> 2 ts_control1/1
  2 ts_control2/1 -> Discrete Derivative/1  "SE_Derivative"
  SE/1 -> 2 ts_control2/1
  Current/1 -> 2 ts_control/1
  2 ts_control/1 -> Bus Creator/1  "Current"

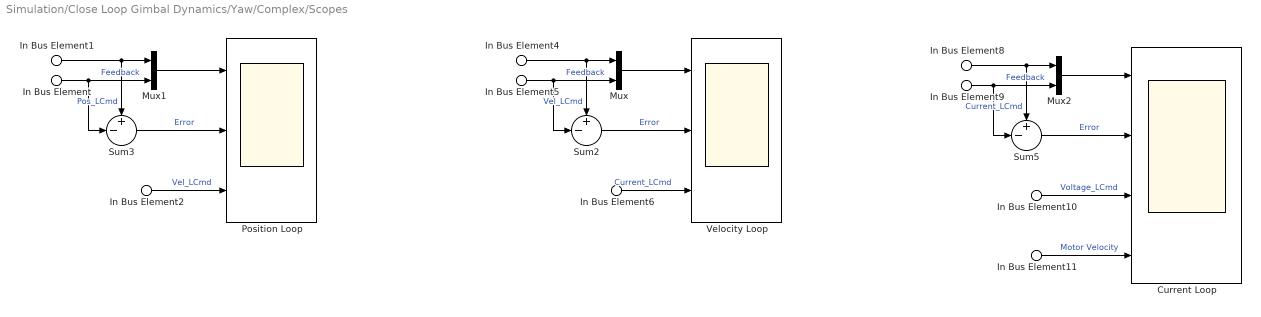
== system Simulation/Close Loop Gimbal Dynamics/Yaw/Complex/Scopes ==
  In Bus Element : Inport  PortName=ScopeSignals  Element=Position.Gyro_Integral
  In Bus Element1 : Inport  PortName=ScopeSignals  Element=Position.Pos_LCmd
  In Bus Element2 : Inport  PortName=ScopeSignals  Element=Position.Vel_LCmd
  In Bus Element4 : Inport  PortName=ScopeSignals  Element=Velocity.Vel_LCmd
  In Bus Element5 : Inport  PortName=ScopeSignals  Element=Velocity.SE_Derivative
  In Bus Element6 : Inport  PortName=ScopeSignals  Element=Velocity.Current_LCmd
  In Bus Element8 : Inport  PortName=ScopeSignals  Element=Current.Current_LCmd
  In Bus Element9 : Inport  PortName=ScopeSignals  Element=Current.Current
  In Bus Element10 : Inport  PortName=ScopeSignals  Element=Current.Voltage_LCmd
  In Bus Element11 : Inport  PortName=ScopeSignals  Element=Current.SE_Derivative
  Current Loop : Scope  NumInputPorts=4
  Mux : Mux  Inputs=2
  Mux1 : Mux  Inputs=2
  Mux2 : Mux  Inputs=2
  Position Loop : Scope  NumInputPorts=3
  Sum2 : Sum  Inputs=+-|
  Sum3 : Sum  Inputs=+-|
  Sum5 : Sum  Inputs=+-|
  Velocity Loop : Scope  NumInputPorts=3
  wires:
  In Bus Element/1 -> Sum3/2, Mux1/2  "Feedback"
  In Bus Element8/1 -> Sum5/1, Mux2/1  "Current_LCmd"
  Sum5/1 -> Current Loop/2  "Error"
  In Bus Element10/1 -> Current Loop/3  "Voltage_LCmd"
  In Bus Element2/1 -> Position Loop/3  "Vel_LCmd"
  Mux2/1 -> Current Loop/1
  In Bus Element9/1 -> Sum5/2, Mux2/2  "Feedback"
  In Bus Element11/1 -> Current Loop/4  "Motor Velocity"
  In Bus Element5/1 -> Sum2/2, Mux/2  "Feedback"
  In Bus Element1/1 -> Sum3/1, Mux1/1  "Pos_LCmd"
  Mux/1 -> Velocity Loop/1
  In Bus Element6/1 -> Velocity Loop/3  "Current_LCmd"
  Mux1/1 -> Position Loop/1
  Sum3/1 -> Position Loop/2  "Error"
  In Bus Element4/1 -> Sum2/1, Mux/1  "Vel_LCmd"
  Sum2/1 -> Velocity Loop/2  "Error"

== system Simulation/Close Loop Gimbal Dynamics/Yaw/Simple/Closed Vel Loop ==
  Relative_w_cmd : Inport
  Closed Vel Loop1 : TransferFcn  Denominator=[1/(2*pi*15) 1]
  Closed Vel Loop2 : Integrator
  Gain : Gain  Gain=db2mag(42)
  Motor2Load : Gain  Gain=1/plant_N
  Sum2 : Sum  Inputs=|+-
  Relative_w : Outport
  wires:
  Relative_w_cmd/1 -> Motor2Load/1
  Motor2Load/1 -> Sum2/1
  Closed Vel Loop1/1 -> Closed Vel Loop2/1
  Closed Vel Loop2/1 -> Relative_w/1, Sum2/2  "Relative_w"
  Sum2/1 -> Gain/1
  Gain/1 -> Closed Vel Loop1/1
